simulink model "sldemo_eml_galaxy"  (Simulink 8.4)
settings: Solver=FixedStepDiscrete  StartTime=0.0  StopTime=250  FixedStep=1  RelTol=1e-3
StartFcn:
  | % Close the plotted figure whe closing the model
  | 
  | foundFig=findobj('Tag','galaxyScreen');
  | 
  | if ishghandle( foundFig ,'figure')
  |    delete(foundFig);
  | end
  | 
  | clear foundFig;
Description:
  | Spiral Galaxy Formation Simulation with MATLAB Function Blocks
  | 
  | This model was inspired by the classic paper "Galactic Bridges and Tails"
  | (Toomre & Toomre 1972). The original paper explained how disc shaped
  | galaxies could develop spiral arms.
  | 
  | Two disc shape galaxies originally are far apart. They then fly by each other
  | and almost collide. Once the galaxies are close enough, mutual gravitational
  | forces cause spiral arms to form.
  | 
  | Except for the "PlotAll" visualization block's use of plotting routines,
  | all MATLAB function blocks in this model support code generation
  | with Simulink Coder(TM) and Embedded Coder(TM).
  | 
  | * Demo Requirements:
  | During this demonstration, Simulink generates code for the simulation in a Simulink
  | project directory created in the current working directory (pwd). If you do not want
  | to affect the current directory (or if you cannot generate files in this directory), you
  | should change your working directory.
CloseFcn:
  | % Close the plotted figure whe closing the model
  | 
  | foundFig=findobj('Tag','galaxyScreen');
  | 
  | if ishghandle( foundFig ,'figure')
  |    delete(foundFig);
  | end
  | 
  | clear foundFig;
settings Model: Creator=The MathWorks Inc.  LastModifiedBy=GM  ExtModeAutoUpdateStatusClock=off
settings DataIOCC: LimitDataPoints=off  SignalLoggingSaveFormat=Dataset  SaveOutput=off  SaveTime=off  SignalLoggingName=sldemo_eml_galaxy_output
settings OptimizationCC: InitFltsAndDblsToZero=on  BufferReusableBoundary=off
settings DebuggingCC: SaveWithParameterizedLinksMsg=none  CheckExecutionContextPreStartOutputMsg=on  CheckExecutionContextRuntimeOutputMsg=on  SignalResolutionControl=TryResolveAllWithWarning  MultiTaskDSMMsg=warning  MultiTaskCondExecSysMsg=none  BusObjectLabelMismatch=none
settings SFSimCC: SFSimOverflowDetection=off  SimParseCustomCode=off
settings RTWCC: IncludeERTFirstTime=on
settings GRTTargetCC: TargetFcnLib=ansi_tfl_tmw.mat

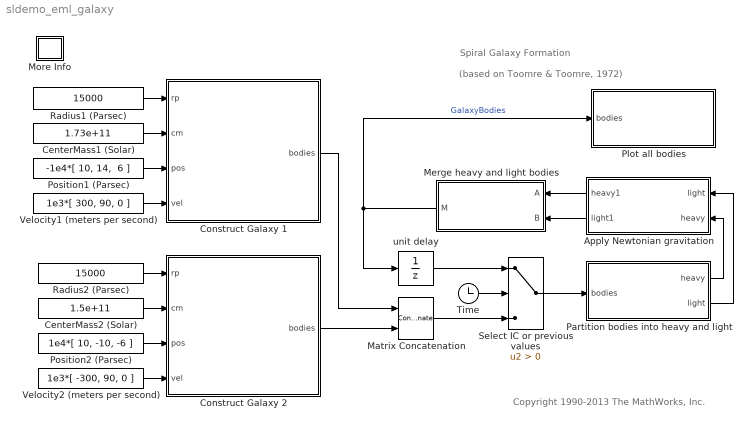
== system sldemo_eml_galaxy ==
  note: Spiral Galaxy Formation
  note: Copyright 1990-2013 The MathWorks, Inc.
  note: (based on Toomre & Toomre, 1972)
  Apply Newtonian gravitation : MATLAB Function  TreatAsAtomicUnit=on
  CenterMass1 (Solar) : Constant  Value=1.73e+11
  CenterMass2 (Solar) : Constant  Value=1.5e+11
  Construct Galaxy 1 : MATLAB Function  TreatAsAtomicUnit=on
  Construct Galaxy 2 : MATLAB Function  TreatAsAtomicUnit=on
  Matrix Concatenation : Concatenate  Mode=Multidimensional array
  Merge heavy and light bodies : MATLAB Function  TreatAsAtomicUnit=on
  More Info : Subsystem
      settings: OpenFcn=showdemo([bdroot(gcs) '_script'])
      mask Display: disp('?')
  Partition bodies into heavy and light : MATLAB Function  TreatAsAtomicUnit=on
  Plot all bodies : MATLAB Function  TreatAsAtomicUnit=on
  Position1 (Parsec) : Constant  Value="-1e4*[ 10, 14,  6 ]"
  Position2 (Parsec) : Constant  Value=1e4*[ 10, -10, -6 ]
  Radius1 (Parsec) : Constant  Value=15000
  Radius2 (Parsec) : Constant  Value=15000
  Select IC or previous values : Switch  Criteria=u2 > Threshold  ZeroCross=off
  Time : Clock
  Velocity1 (meters per second) : Constant  Value=1e3*[ 300, 90, 0 ]
  Velocity2 (meters per second) : Constant  Value=1e3*[ -300, 90, 0 ]
  unit delay : UnitDelay  SampleTime=-1
  wires:
  Radius1 (Parsec)/1 -> Construct Galaxy 1/1(rp)
  CenterMass1 (Solar)/1 -> Construct Galaxy 1/2(cm)
  Apply Newtonian gravitation/1(heavy1) -> Merge heavy and light bodies/1(A)
  Apply Newtonian gravitation/2(light1) -> Merge heavy and light bodies/2(B)
  Merge heavy and light bodies/1(M) -> unit delay/1, Plot all bodies/1(bodies)  "GalaxyBodies"
  Time/1 -> Select IC or previous values/2
  Select IC or previous values/1 -> Partition bodies into heavy and light/1(bodies)
  unit delay/1 -> Select IC or previous values/1
  Position1 (Parsec)/1 -> Construct Galaxy 1/3(pos)
  Velocity1 (meters per second)/1 -> Construct Galaxy 1/4(vel)
  Radius2 (Parsec)/1 -> Construct Galaxy 2/1(rp)
  CenterMass2 (Solar)/1 -> Construct Galaxy 2/2(cm)
  Position2 (Parsec)/1 -> Construct Galaxy 2/3(pos)
  Velocity2 (meters per second)/1 -> Construct Galaxy 2/4(vel)
  Matrix Concatenation/1 -> Select IC or previous values/3
  Partition bodies into heavy and light/1(heavy) -> Apply Newtonian gravitation/2(heavy)
  Construct Galaxy 1/1(bodies) -> Matrix Concatenation/1
  Construct Galaxy 2/1(bodies) -> Matrix Concatenation/2
  Partition bodies into heavy and light/2(light) -> Apply Newtonian gravitation/1(light)

== system sldemo_eml_galaxy/More Info ==

== matlab function Plot all bodies ==
  data: bodies input double
function PlotAll(bodies)

persistent fig;
persistent oldPlot;

coder.extrinsic('findobj','get','set','figure','clf','hold','text','delete','plot3','drawnow');

n = size(bodies,1);

SpeedOfLight = 299792458; % in m/s
YearInSeconds = 365*24*60*60;
LightYear = SpeedOfLight*YearInSeconds;
Parsec = 3.26*LightYear;
foundFig = findobj('Tag','galaxyScreen');

if isempty(fig)||isempty(foundFig)
    if isempty(foundFig)
        fig = figure;
    else
        fig = figure(foundFig);
    end;
    clf(fig);
    set(fig, 'Name', 'Galaxy');
    set(fig, 'Tag', 'galaxyScreen');
    set(fig, 'Renderer', 'painters');
    set(fig, 'Color', 'black');
    hold('on');
    fig_axes = get(fig, 'CurrentAxes');
    init_axes(fig_axes);
    text(0,3.5*30000*Parsec,0,...
        ['Spiral galaxy formation on close encounters', ...
        char(10),'(based on Toomre & Toomre, 1972)'],...
        'Color','green','FontSize',12, 'HorizontalAlignment','center');
end

points_x = zeros(1,n);
points_y = zeros(1,n);
points_z = zeros(1,n);
points_col = zeros(1,n);
for i = 1:n,
    points_x(i) = bodies(i,2);
    points_y(i) = bodies(i,3);
    points_z(i) = bodies(i,4);
    points_col(i) = bodies(i,8);
end

%
% Remove the old plot.
%
if isempty(oldPlot)
    oldPlot = fig;
elseif ~isempty(foundFig)
    delete(oldPlot);
end

oldPlot = plot3(points_x,points_y,points_z,'w.');
drawnow;

function init_axes(a)

coder.extrinsic('set');

SpeedOfLight = 299792458; % in m/s
YearInSeconds = 365*24*60*60;
LightYear = SpeedOfLight*YearInSeconds;
Parsec = 3.26*LightYear;
set(a, 'CameraTarget', [0,0,0] );
set(a, 'CameraPosition', [0,22000*Parsec*3,18000*Parsec*3]);
set(a, 'CameraViewAngle', 80 );
set(a, 'CameraUpVector', [0,1,0]);
set(a, 'Visible', 'off' );
set(a, 'XLim', [-25000*Parsec*8,30000*Parsec*8]);
set(a, 'YLim', [-25000*Parsec*8,30000*Parsec*8]);
set(a, 'ZLim', [-30000*Parsec*8,30000*Parsec*8]);

== matlab function Construct Galaxy 1 ==
  data: rp input double; cm input double; bodies output double; pos input double; vel input double
function bodies = ConstructGalaxy(rp,cm,pos,vel)

persistent bs;
numberOfBodies = 350;

if isempty(bs);
    rng('default');
    bs = ConstructGalaxy0(rp,cm,pos,vel,numberOfBodies);
end

bodies = bs;

function bodies = ConstructGalaxy0(rp,cm,pos,vel,n)

SolarMass = 1.9891e+30; % In kg
G = 6.672E-11; % Nm^2/kg^2 (Gravitational constant)
SpeedOfLight = 299792458; % in m/s
YearInSeconds = 365*24*60*60;
LightYear = SpeedOfLight*YearInSeconds;
Parsec = 3.26*LightYear;

radiusOuter = rp*Parsec;
radiusInner = (rp/3)*Parsec;

% Each star has X,Y,Z,VX,VY,VZ
% X,Y,Z position in cartesian coordinates
% VX,VY,VZ velocity in cartesian coordinates
cm = cm*SolarMass;

bodies = zeros(n,8);
bodies(1,1) = cm;
bodies(1,2) = pos(1)*Parsec;
bodies(1,3) = pos(2)*Parsec;
bodies(1,4) = pos(3)*Parsec;
bodies(1,5) = vel(1);
bodies(1,6) = vel(2);
bodies(1,7) = vel(3);
bodies(1,8) = 'r';

if n > 1
    for i = 2:n,
        m0 = rand*20+4;
        m = m0*SolarMass;
        r = rand*(radiusOuter - radiusInner) + radiusInner;
        arg = rand*(2*pi);
        x = r*cos(arg);
        y = r*sin(arg);
        z = 0;
        dx = cos(arg+pi/2);
        dy = sin(arg+pi/2);
        dz = 0;
        % Compute free fall velocity
        v = sqrt(G*cm/r);
        bodies(i,1) = m;
        bodies(i,2) = x+pos(1)*Parsec;
        bodies(i,3) = y+pos(2)*Parsec;
        bodies(i,4) = z+pos(3)*Parsec;
        bodies(i,5) = dx*v+vel(1);
        bodies(i,6) = dy*v+vel(2);
        bodies(i,7) = dz*v+vel(3);
        bodies(i,8) = 'r';
    end
end

== matlab function Apply Newtonian gravitation ==
  data: heavy1 output double; light1 output double; light input double; heavy input double
function [heavy1,light1] = ApplyGravity(light,heavy)

G = 6.672E-11; % Nm^2/kg^2 (Gravitational constant)

YearInSeconds = 365*24*60*60;
timeStep = 2000000*YearInSeconds;

n = size(heavy,1);

heavy1 = heavy;
light1 = light;

for i = 1:n,
    mi = heavy(i,1);
    if mi == 0
        break;
    end
    xi = heavy(i,2);
    yi = heavy(i,3);
    zi = heavy(i,4);
    ar = [0 0 0];
    for j = 1:n,
        if i ~= j,
            mj = heavy(j,1);
            if mj == 0
                break;
            end
            xj = heavy(j,2);
            yj = heavy(j,3);
            zj = heavy(j,4);
            d = [xj yj zj] - [xi yi zi];
            dr2 = d(1)*d(1)+d(2)*d(2)+d(3)*d(3);
            ar = ar + (d/sqrt(dr2))*((G*mj)/dr2);
        end
    end
    for k = 1:3
        heavy1(i,4+k) = heavy(i,4+k) + ar(k)*timeStep;
    end
end

for i = 1:n,
    mi = light(i,1);
    if mi == 0
        break;
    end
    xi = light(i,2);
    yi = light(i,3);
    zi = light(i,4);
    ar = [0 0 0];
    for j = 1:n,
        mj = heavy(j,1);
        if mj == 0
            break;
        end
        xj = heavy(j,2);
        yj = heavy(j,3);
        zj = heavy(j,4);
        d = [xj yj zj] - [xi yi zi];
        dr2 = d(1)*d(1)+ d(2)*d(2) + d(3)*d(3);
        ar = ar + (d/sqrt(dr2))*((G*mj)/dr2);
    end
    for k = 1:3
        light1(i,4+k) = light(i,4+k) + ar(k)*timeStep;
    end
end

for i = 1:n
    for k = 1:3
        heavy1(i,k+1) = heavy1(i,k+1) + timeStep*heavy1(i,k+4);
    end
    for k = 1:3
        light1(i,k+1) = light1(i,k+1) + timeStep*light1(i,k+4);
    end
end

== matlab function Partition bodies into heavy and light ==
  data: bodies input double; heavy output double; light output double
function [heavy,light] = Partition(bodies)

SolarMass = 1.9891e+30; % kg
Limit = 100*SolarMass;

n = size(bodies,1);
props = size(bodies,2);
heavy = zeros(n,props);
light = zeros(n,props);

lightIndex = 1;
heavyIndex = 1;

for i = 1:n
    m = bodies(i,1);
    if m < Limit
        light(lightIndex,:) = bodies(i,:);
        lightIndex = lightIndex + 1;
    else
        heavy(heavyIndex,:) = bodies(i,:);
        heavyIndex = heavyIndex + 1;
    end
end

== matlab function Merge heavy and light bodies ==
  data: A input double; B input double; M output double
function M = combine(A,B)

n = size(A,1);
nProps = size(A,2);
M = zeros(n,nProps);
for i = 1:n
    if A(i,1) == 0
        break
    end
    M(i,:) = A(i,:);
end
n1 = n - i + 1;
for j = 1:n1
    M(j+i-1,:) = B(j,:);
    if B(i,1) == 0
        break
    end
end

== matlab function Construct Galaxy 2 ==
  data: rp input double; cm input double; bodies output double; pos input double; vel input double
function bodies = ConstructGalaxy(rp,cm,pos,vel)

persistent bs;
numberOfBodies = 350;

if isempty(bs);
    rng('default');
    bs = ConstructGalaxy0(rp,cm,pos,vel,numberOfBodies);
end

bodies = bs;

function bodies = ConstructGalaxy0(rp,cm,pos,vel,n)

SolarMass = 1.9891e+30; % In kg
G = 6.672E-11; % Nm^2/kg^2 (Gravitational constant)
SpeedOfLight = 299792458; % in m/s
YearInSeconds = 365*24*60*60;
LightYear = SpeedOfLight*YearInSeconds;
Parsec = 3.26*LightYear;

radiusOuter = rp*Parsec;
radiusInner = (rp/3)*Parsec;

% Each star has X,Y,Z,VX,VY,VZ
% X,Y,Z position in certesian coordinates
% VX,VY,VZ velocity in certesian coordinates
cm = cm*SolarMass;

bodies = zeros(n,8);
bodies(1,1) = cm;
bodies(1,2) = pos(1)*Parsec;
bodies(1,3) = pos(2)*Parsec;
bodies(1,4) = pos(3)*Parsec;
bodies(1,5) = vel(1);
bodies(1,6) = vel(2);
bodies(1,7) = vel(3);
bodies(1,8) = 'y';

if n > 1
    for i = 2:n,
        m0 = rand*20+4;
        m = m0*SolarMass;
        r = rand*(radiusOuter - radiusInner) + radiusInner;
        arg = rand*(2*pi);
        x = r*cos(arg);
        y = r*sin(arg);
        z = 0;
        dx = cos(arg+pi/2);
        dy = sin(arg+pi/2);
        dz = 0;
        % Compute free fall velocity
        v = sqrt(G*cm/r);
        bodies(i,1) = m;
        bodies(i,2) = x+pos(1)*Parsec;
        bodies(i,3) = y+pos(2)*Parsec;
        bodies(i,4) = z+pos(3)*Parsec;
        bodies(i,5) = dx*v+vel(1);
        bodies(i,6) = dy*v+vel(2);
        bodies(i,7) = dz*v+vel(3);
        bodies(i,8) = 'y';
    end
end
